simulink model "ue_1_a"  (R2015b)
settings: Solver=VariableStepAuto  StartTime=0.0  StopTime=100.0  RelTol=1e-3
settings Model: Creator=dbarelop  LastModifiedBy=dbarelop

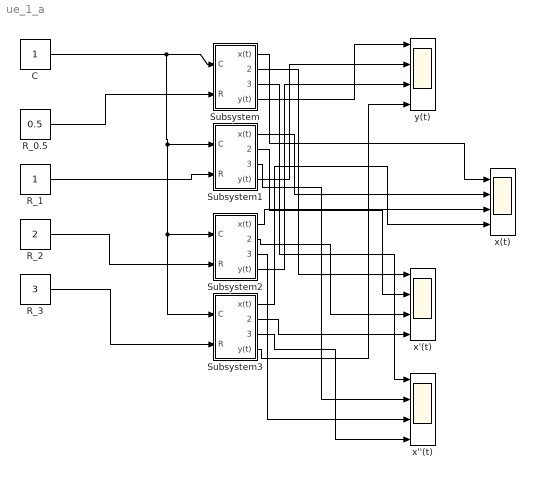
== system ue_1_a ==
  C : Constant
  R_0.5 : Constant  Value=0.5
  R_1 : Constant
  R_2 : Constant  Value=2
  R_3 : Constant  Value=3
  Subsystem : Subsystem
  Subsystem1 : Subsystem
  Subsystem2 : Subsystem
  Subsystem3 : Subsystem
  x''(t) : Scope  NumInputPorts=4
  x'(t) : Scope  NumInputPorts=4
  x(t) : Scope  NumInputPorts=4
  y(t) : Scope  NumInputPorts=4
  wires:
  R_0.5/1 -> Subsystem/2(R)
  R_3/1 -> Subsystem3/2(R)
  Subsystem/1(x(t)) -> x(t)/1
  Subsystem/2(x'(t)) -> x'(t)/1
  Subsystem/3(x''(t)) -> x''(t)/1
  Subsystem1/1(x(t)) -> x(t)/2
  Subsystem1/2(x'(t)) -> x'(t)/2
  Subsystem1/3(x''(t)) -> x''(t)/2
  Subsystem2/1(x(t)) -> x(t)/3
  Subsystem2/2(x'(t)) -> x'(t)/3
  Subsystem3/1(x(t)) -> x(t)/4
  Subsystem3/2(x'(t)) -> x'(t)/4
  Subsystem2/3(x''(t)) -> x''(t)/3
  Subsystem3/3(x''(t)) -> x''(t)/4
  Subsystem/4(y(t)) -> y(t)/1
  R_1/1 -> Subsystem1/2(R)
  Subsystem1/4(y(t)) -> y(t)/2
  C/1 -> Subsystem1/1(C), Subsystem3/1(C), Subsystem2/1(C), Subsystem/1(C)
  R_2/1 -> Subsystem2/2(R)
  Subsystem2/4(y(t)) -> y(t)/3
  Subsystem3/4(y(t)) -> y(t)/4

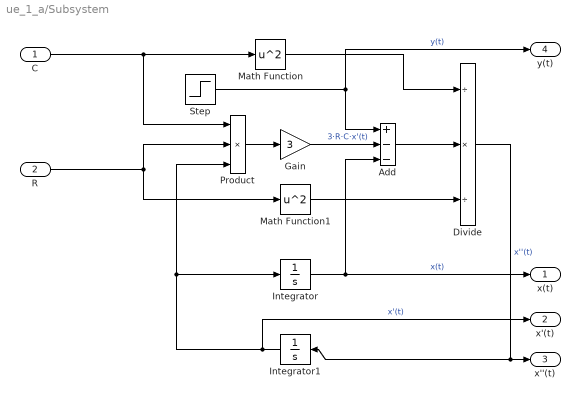
== system ue_1_a/Subsystem ==
  C : Inport
  R : Inport  Port=2
  Add : Sum  Inputs=+--
  Divide : Product  Inputs=/*/
  Gain : Gain  Gain=3
  Integrator : Integrator
  Integrator1 : Integrator
  Math Function : Math  Operator=square  SaturateOnIntegerOverflow=on
  Math Function1 : Math  Operator=square  SaturateOnIntegerOverflow=on
  Product : Product  Inputs=3
  Step : Step  SampleTime=0
  x(t) : Outport
  x'(t) : Outport  Port=2
  x''(t) : Outport  Port=3
  y(t) : Outport  Port=4
  wires:
  Add/1 -> Divide/2
  C/1 -> Product/1, Math Function/1
  Math Function/1 -> Divide/1
  Math Function1/1 -> Divide/3
  Divide/1 -> Integrator1/1, x''(t)/1  "x''(t)"
  Integrator1/1 -> x'(t)/1, Product/3, Integrator/1  "x'(t)"
  Step/1 -> Add/1, y(t)/1  "y(t)"
  R/1 -> Product/2, Math Function1/1
  Product/1 -> Gain/1
  Integrator/1 -> x(t)/1, Add/3  "x(t)"
  Gain/1 -> Add/2  "3·R·C·x'(t)"

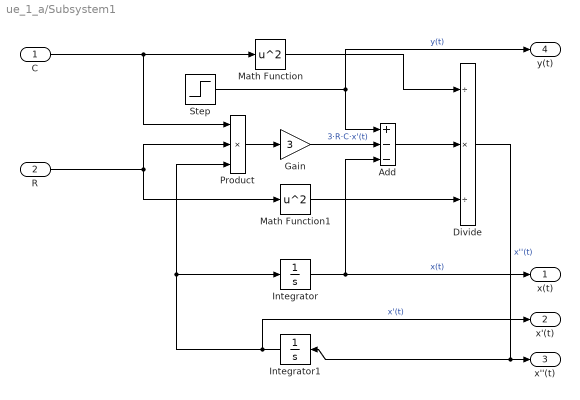
== system ue_1_a/Subsystem1 ==
  C : Inport
  R : Inport  Port=2
  Add : Sum  Inputs=+--
  Divide : Product  Inputs=/*/
  Gain : Gain  Gain=3
  Integrator : Integrator
  Integrator1 : Integrator
  Math Function : Math  Operator=square  SaturateOnIntegerOverflow=on
  Math Function1 : Math  Operator=square  SaturateOnIntegerOverflow=on
  Product : Product  Inputs=3
  Step : Step  SampleTime=0
  x(t) : Outport
  x'(t) : Outport  Port=2
  x''(t) : Outport  Port=3
  y(t) : Outport  Port=4
  wires:
  Add/1 -> Divide/2
  C/1 -> Product/1, Math Function/1
  Math Function/1 -> Divide/1
  Math Function1/1 -> Divide/3
  Divide/1 -> Integrator1/1, x''(t)/1  "x''(t)"
  Integrator1/1 -> x'(t)/1, Product/3, Integrator/1  "x'(t)"
  Step/1 -> Add/1, y(t)/1  "y(t)"
  R/1 -> Product/2, Math Function1/1
  Product/1 -> Gain/1
  Integrator/1 -> x(t)/1, Add/3  "x(t)"
  Gain/1 -> Add/2  "3·R·C·x'(t)"

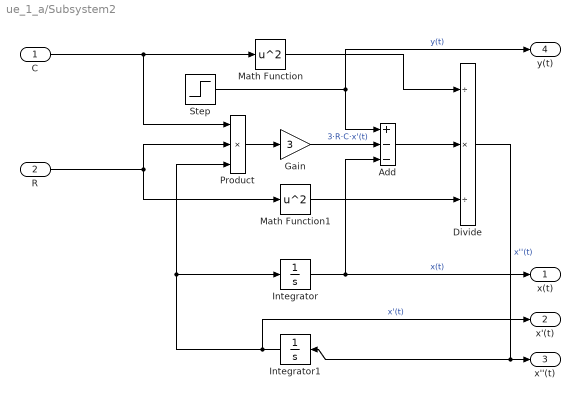
== system ue_1_a/Subsystem2 ==
  C : Inport
  R : Inport  Port=2
  Add : Sum  Inputs=+--
  Divide : Product  Inputs=/*/
  Gain : Gain  Gain=3
  Integrator : Integrator
  Integrator1 : Integrator
  Math Function : Math  Operator=square  SaturateOnIntegerOverflow=on
  Math Function1 : Math  Operator=square  SaturateOnIntegerOverflow=on
  Product : Product  Inputs=3
  Step : Step  SampleTime=0
  x(t) : Outport
  x'(t) : Outport  Port=2
  x''(t) : Outport  Port=3
  y(t) : Outport  Port=4
  wires:
  Add/1 -> Divide/2
  C/1 -> Product/1, Math Function/1
  Math Function/1 -> Divide/1
  Math Function1/1 -> Divide/3
  Divide/1 -> Integrator1/1, x''(t)/1  "x''(t)"
  Integrator1/1 -> x'(t)/1, Product/3, Integrator/1  "x'(t)"
  Step/1 -> Add/1, y(t)/1  "y(t)"
  R/1 -> Product/2, Math Function1/1
  Product/1 -> Gain/1
  Integrator/1 -> x(t)/1, Add/3  "x(t)"
  Gain/1 -> Add/2  "3·R·C·x'(t)"

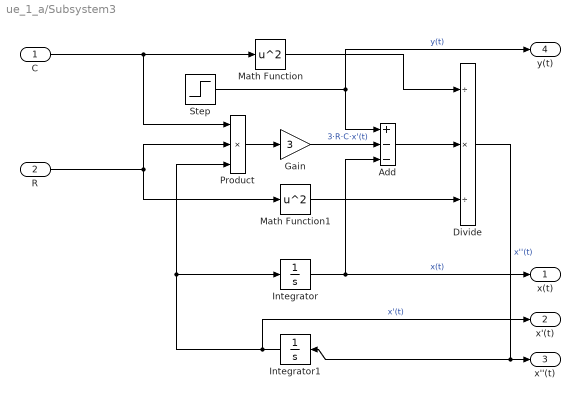
== system ue_1_a/Subsystem3 ==
  C : Inport
  R : Inport  Port=2
  Add : Sum  Inputs=+--
  Divide : Product  Inputs=/*/
  Gain : Gain  Gain=3
  Integrator : Integrator
  Integrator1 : Integrator
  Math Function : Math  Operator=square  SaturateOnIntegerOverflow=on
  Math Function1 : Math  Operator=square  SaturateOnIntegerOverflow=on
  Product : Product  Inputs=3
  Step : Step  SampleTime=0
  x(t) : Outport
  x'(t) : Outport  Port=2
  x''(t) : Outport  Port=3
  y(t) : Outport  Port=4
  wires:
  Add/1 -> Divide/2
  C/1 -> Product/1, Math Function/1
  Math Function/1 -> Divide/1
  Math Function1/1 -> Divide/3
  Divide/1 -> Integrator1/1, x''(t)/1  "x''(t)"
  Integrator1/1 -> x'(t)/1, Product/3, Integrator/1  "x'(t)"
  Step/1 -> Add/1, y(t)/1  "y(t)"
  R/1 -> Product/2, Math Function1/1
  Product/1 -> Gain/1
  Integrator/1 -> x(t)/1, Add/3  "x(t)"
  Gain/1 -> Add/2  "3·R·C·x'(t)"
